simulink model "discreto"  (Simulink 5.0)
settings: Solver=ode3  StartTime=0.0  StopTime=TMAX  FixedStep=Ta  RelTol=1e-3
values from neighbouring files (symbols this model uses):
  A = [-1/p                0                  1 ... (first row only)    [script_controle_lr.m]    (also in scriptdiscreto.m = 30)
  den = Gz.Den{1}    [scriptdiscreto.m]
  Kd = 0.0101    [scriptdiscreto.m]
  Ki = 0.1882    [scriptdiscreto.m]
  Kp = 0.0618    [scriptdiscreto.m]
  LOWER_SAT = -5    [scriptdiscreto.m]
  MEDIA_RUIDO = 0    [scriptdiscreto.m]
  num = Gz.Num{1}    [scriptdiscreto.m]
  Ta = 0.2    [discretizacao.m]    (also in scriptdiscreto.m = 0.001)
  teta = 0    [scriptdiscreto.m]
  UPPER_SAT = 5    [scriptdiscreto.m]
  VARIANCIA_RUIDO = 0.05    [scriptdiscreto.m]
settings Model: LastModifiedBy=ENGENHARIA

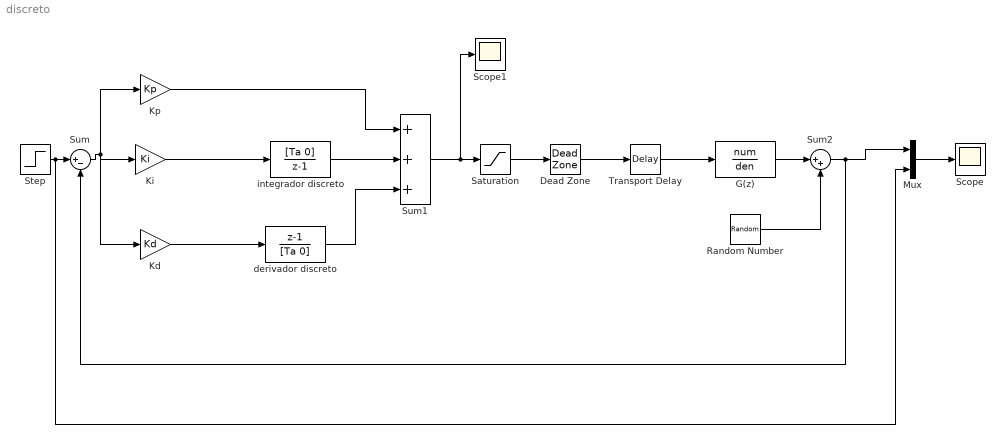
== system discreto ==
  Dead Zone : DeadZone  LowerValue=START_DEAD_ZONE  UpperValue=END_DEAD_ZONE  SaturateOnIntegerOverflow=on
  G(z) : DiscreteTransferFcn  Numerator=num  Denominator=den  SampleTime=Ta
  Kd : Gain  Gain=Kd  SaturateOnIntegerOverflow=on
  Ki : Gain  Gain=Ki  SaturateOnIntegerOverflow=on
  Kp : Gain  Gain=Kp  SaturateOnIntegerOverflow=on
  Mux : Mux  Inputs=2
  Random Number : RandomNumber  Mean=MEDIA_RUIDO  Variance=VARIANCIA_RUIDO  SampleTime=0
  Saturation : Saturate  UpperLimit=UPPER_SAT  LowerLimit=LOWER_SAT
  Scope : Scope
      settings: TimeRange=10  SaveName=sinais  DataFormat=Array
  Scope1 : Scope
      settings: TimeRange=10  YMin=-1
  Step : Step  Time=0  After=A  SampleTime=0
  Sum : Sum  Inputs=|+-  SaturateOnIntegerOverflow=on
  Sum1 : Sum  Inputs=+++  SaturateOnIntegerOverflow=on
  Sum2 : Sum  Inputs=|++  SaturateOnIntegerOverflow=on
  Transport Delay : TransportDelay  DelayTime=teta
  derivador discreto : DiscreteTransferFcn  Numerator=[1 -1]  Denominator=[Ta 0]  SampleTime=Ta
  integrador discreto : DiscreteTransferFcn  Numerator=[Ta 0]  Denominator="[1  -1]"  SampleTime=Ta
  wires:
  Saturation/1 -> Dead Zone/1
  Dead Zone/1 -> Transport Delay/1
  Step/1 -> Sum/1, Mux/2
  Kp/1 -> Sum1/1
  integrador discreto/1 -> Sum1/2
  Ki/1 -> integrador discreto/1
  Kd/1 -> derivador discreto/1
  Sum/1 -> Kp/1, Kd/1, Ki/1
  Sum1/1 -> Saturation/1, Scope1/1
  Mux/1 -> Scope/1
  G(z)/1 -> Sum2/1
  Random Number/1 -> Sum2/2
  Sum2/1 -> Mux/1, Sum/2
  derivador discreto/1 -> Sum1/3
  Transport Delay/1 -> G(z)/1
